simulink model "Stromsensor_three_fase"  (R2020b)
settings: Solver=VariableStepAuto  StartTime=0.0  StopTime=1/60*2  RelTol=1e-3
libraries: fl_lib x27, nesl_utility x9, ee_lib x3
settings Model: Creator=jenel  LastModifiedBy=jenel

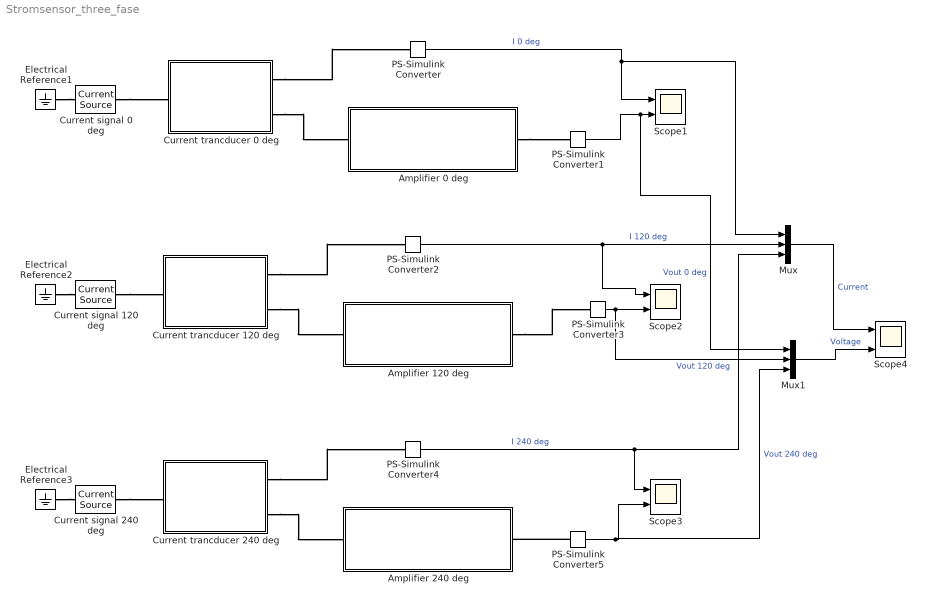
== system Stromsensor_three_fase ==
  Amplifier 0 deg : Subsystem
  Amplifier 120 deg : Subsystem
  Amplifier 240 deg : Subsystem
  Current signal 0 deg : ee_lib/Sources/Current Source  dc_current=0 A  ac_current=200 mA  ac_shift=0 deg  ac_frequency=60 Hz  noise_mode=0  PSD=0 A^2/Hz  repeatability=1  auto_seed=961264961  user_seed=0  sample_time=1e-3 s  i_specify=off  i_priority=None  i=0 A  i_nominal_specify=off  i_nominal_unit=A  i_nominal_value=1  v_specify=off  v_priority=None  v=0 V  v_nominal_specify=off  v_nominal_unit=V  v_nominal_value=1
      settings: SourceProductBaseCode=PS
  Current signal 120 deg : ee_lib/Sources/Current Source  dc_current=0 A  ac_current=200 mA  ac_shift=120 deg  ac_frequency=60 Hz  noise_mode=0  PSD=0 A^2/Hz  repeatability=1  auto_seed=3499211588  user_seed=0  sample_time=1e-3 s  i_specify=off  i_priority=None  i=0 A  i_nominal_specify=off  i_nominal_unit=A  i_nominal_value=1  v_specify=off  v_priority=None  v=0 V  v_nominal_specify=off  v_nominal_unit=V  v_nominal_value=1
      settings: SourceProductBaseCode=PS
  Current signal 240 deg : ee_lib/Sources/Current Source  dc_current=0 A  ac_current=200 mA  ac_shift=240 deg  ac_frequency=60 Hz  noise_mode=0  PSD=0 A^2/Hz  repeatability=1  auto_seed=3890346746  user_seed=0  sample_time=1e-3 s  i_specify=off  i_priority=None  i=0 A  i_nominal_specify=off  i_nominal_unit=A  i_nominal_value=1  v_specify=off  v_priority=None  v=0 V  v_nominal_specify=off  v_nominal_unit=V  v_nominal_value=1
      settings: SourceProductBaseCode=PS
  Current trancducer 0 deg : Subsystem
  Current trancducer 120 deg : Subsystem
  Current trancducer 240 deg : Subsystem
  Electrical Reference1 : fl_lib/Electrical/Electrical Elements/Electrical Reference
  Electrical Reference2 : fl_lib/Electrical/Electrical Elements/Electrical Reference
  Electrical Reference3 : fl_lib/Electrical/Electrical Elements/Electrical Reference
  Mux : Mux  Inputs=3
  Mux1 : Mux  Inputs=3
  PS-Simulink Converter{,1..5} (6 alike) : nesl_utility/PS-Simulink Converter  PhysicalDomain=network_engine_domain  SubClassName=ps_output  LeftPortType=input  RightPortType=output  PseudoPeriodic=off  Frequencies=[]  Unit=inherit  AffineConversion=off
  Scope{1..4} (4 alike) : Scope  NumInputPorts=2
  wires:
  PS-Simulink Converter/1 -> Mux/1, Scope1/1  "I 0 deg"
  PS-Simulink Converter1/1 -> Mux1/1, Scope1/2  "Vout 0 deg"
  PS-Simulink Converter3/1 -> Mux1/2, Scope2/2  "Vout 120 deg"
  PS-Simulink Converter2/1 -> Scope2/1, Mux/2  "I 120 deg"
  PS-Simulink Converter4/1 -> Mux/3, Scope3/1  "I 240 deg"
  PS-Simulink Converter5/1 -> Mux1/3, Scope3/2  "Vout 240 deg"
  Mux/1 -> Scope4/1  "Current"
  Mux1/1 -> Scope4/2  "Voltage"
  connections:
  Current trancducer 0 deg/RConn1 -- PS-Simulink Converter/LConn1
  Electrical Reference1/LConn1 -- Current signal 0 deg/RConn1
  Current signal 0 deg/LConn1 -- Current trancducer 0 deg/LConn1
  Current trancducer 0 deg/RConn2 -- Amplifier 0 deg/LConn1
  Amplifier 0 deg/RConn1 -- PS-Simulink Converter1/LConn1
  Current trancducer 120 deg/RConn2 -- Amplifier 120 deg/LConn1
  Current signal 120 deg/LConn1 -- Current trancducer 120 deg/LConn1
  Amplifier 120 deg/RConn1 -- PS-Simulink Converter3/LConn1
  Electrical Reference2/LConn1 -- Current signal 120 deg/RConn1
  Current trancducer 120 deg/RConn1 -- PS-Simulink Converter2/LConn1
  Current trancducer 240 deg/RConn1 -- PS-Simulink Converter4/LConn1
  Electrical Reference3/LConn1 -- Current signal 240 deg/RConn1
  PS-Simulink Converter5/LConn1 -- Amplifier 240 deg/RConn1
  Current signal 240 deg/LConn1 -- Current trancducer 240 deg/LConn1
  Current trancducer 240 deg/RConn2 -- Amplifier 240 deg/LConn1

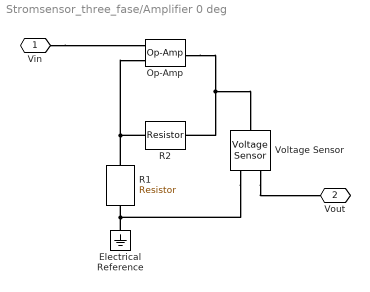
== system Stromsensor_three_fase/Amplifier 0 deg ==
  Electrical Reference : fl_lib/Electrical/Electrical Elements/Electrical Reference
  Op-Amp : fl_lib/Electrical/Electrical Elements/Op-Amp  outI_specify=on  outI_priority=None  outI=0 A  outI_nominal_specify=off  outI_nominal_unit=A  outI_nominal_value=1
  R1 : fl_lib/Electrical/Electrical Elements/Resistor  R=1000 Ohm  i_specify=off  i_priority=None  i=0 A  i_nominal_specify=off  i_nominal_unit=A  i_nominal_value=1  v_specify=off  v_priority=None  v=0 V  v_nominal_specify=off  v_nominal_unit=V  v_nominal_value=1
  R2 : fl_lib/Electrical/Electrical Elements/Resistor  R=666.6667 Ohm  i_specify=off  i_priority=None  i=0 A  i_nominal_specify=off  i_nominal_unit=A  i_nominal_value=1  v_specify=off  v_priority=None  v=0 V  v_nominal_specify=off  v_nominal_unit=V  v_nominal_value=1
  Voltage Sensor : fl_lib/Electrical/Electrical Sensors/Voltage Sensor
  Vin : PMIOPort  Side=Left
  Vout : PMIOPort  Port=2  Side=Right
  connections:
  Op-Amp/RConn1 -- Voltage Sensor/LConn1 -- R2/RConn1
  Vin/RConn1 -- Op-Amp/LConn1
  Electrical Reference/LConn1 -- Voltage Sensor/RConn2 -- R1/RConn1
  R2/LConn1 -- R1/LConn1 -- Op-Amp/LConn2
  Voltage Sensor/RConn1 -- Vout/RConn1

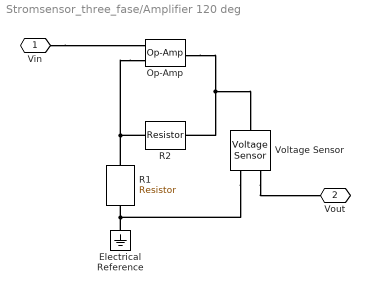
== system Stromsensor_three_fase/Amplifier 120 deg ==
  Electrical Reference : fl_lib/Electrical/Electrical Elements/Electrical Reference
  Op-Amp : fl_lib/Electrical/Electrical Elements/Op-Amp  outI_specify=on  outI_priority=None  outI=0 A  outI_nominal_specify=off  outI_nominal_unit=A  outI_nominal_value=1
  R1 : fl_lib/Electrical/Electrical Elements/Resistor  R=1000 Ohm  i_specify=off  i_priority=None  i=0 A  i_nominal_specify=off  i_nominal_unit=A  i_nominal_value=1  v_specify=off  v_priority=None  v=0 V  v_nominal_specify=off  v_nominal_unit=V  v_nominal_value=1
  R2 : fl_lib/Electrical/Electrical Elements/Resistor  R=666.6667 Ohm  i_specify=off  i_priority=None  i=0 A  i_nominal_specify=off  i_nominal_unit=A  i_nominal_value=1  v_specify=off  v_priority=None  v=0 V  v_nominal_specify=off  v_nominal_unit=V  v_nominal_value=1
  Voltage Sensor : fl_lib/Electrical/Electrical Sensors/Voltage Sensor
  Vin : PMIOPort  Side=Left
  Vout : PMIOPort  Port=2  Side=Right
  connections:
  Voltage Sensor/RConn1 -- Vout/RConn1
  Op-Amp/LConn2 -- R1/LConn1 -- R2/LConn1
  Voltage Sensor/RConn2 -- R1/RConn1 -- Electrical Reference/LConn1
  Vin/RConn1 -- Op-Amp/LConn1
  R2/RConn1 -- Voltage Sensor/LConn1 -- Op-Amp/RConn1

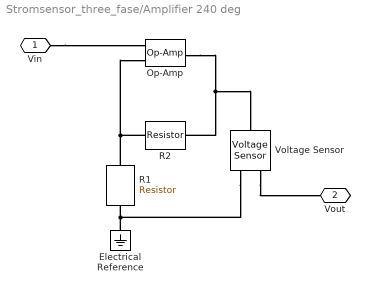
== system Stromsensor_three_fase/Amplifier 240 deg ==
  Electrical Reference : fl_lib/Electrical/Electrical Elements/Electrical Reference
  Op-Amp : fl_lib/Electrical/Electrical Elements/Op-Amp  outI_specify=on  outI_priority=None  outI=0 A  outI_nominal_specify=off  outI_nominal_unit=A  outI_nominal_value=1
  R1 : fl_lib/Electrical/Electrical Elements/Resistor  R=1000 Ohm  i_specify=off  i_priority=None  i=0 A  i_nominal_specify=off  i_nominal_unit=A  i_nominal_value=1  v_specify=off  v_priority=None  v=0 V  v_nominal_specify=off  v_nominal_unit=V  v_nominal_value=1
  R2 : fl_lib/Electrical/Electrical Elements/Resistor  R=666.6667 Ohm  i_specify=off  i_priority=None  i=0 A  i_nominal_specify=off  i_nominal_unit=A  i_nominal_value=1  v_specify=off  v_priority=None  v=0 V  v_nominal_specify=off  v_nominal_unit=V  v_nominal_value=1
  Voltage Sensor : fl_lib/Electrical/Electrical Sensors/Voltage Sensor
  Vin : PMIOPort  Side=Left
  Vout : PMIOPort  Port=2  Side=Right
  connections:
  Op-Amp/RConn1 -- Voltage Sensor/LConn1 -- R2/RConn1
  Vin/RConn1 -- Op-Amp/LConn1
  Electrical Reference/LConn1 -- R1/RConn1 -- Voltage Sensor/RConn2
  R2/LConn1 -- R1/LConn1 -- Op-Amp/LConn2
  Voltage Sensor/RConn1 -- Vout/RConn1

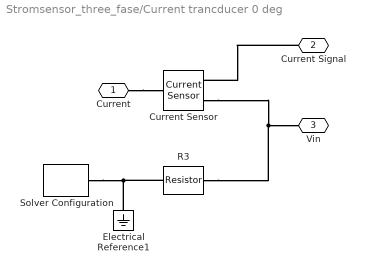
== system Stromsensor_three_fase/Current trancducer 0 deg ==
  Current Sensor : fl_lib/Electrical/Electrical Sensors/Current Sensor
  Electrical Reference1 : fl_lib/Electrical/Electrical Elements/Electrical Reference
  R3 : fl_lib/Electrical/Electrical Elements/Resistor  R=30 Ohm  i_specify=off  i_priority=None  i=0 A  i_nominal_specify=off  i_nominal_unit=A  i_nominal_value=1  v_specify=off  v_priority=None  v=0 V  v_nominal_specify=off  v_nominal_unit=V  v_nominal_value=1
  Solver Configuration : nesl_utility/Solver Configuration  PhysicalDomain=network_engine_domain  SubClassName=solver  LeftPortType=input  RightPortType=generic  Tones=[]  Harmonics=[]  SimulateNoise=off  Profile=off  UseLocalSampling=off  EnableSwitchedLinearOptims=on  FrequencyDomain=off  UseCCode=off  RelTol=0.001  AbsTol=1e-06  MinStep=1e-09  ToWorkspace=off  RevertToSquareIcSolve=off  NumHomotopyIterations=100  PhasorMode=off  PhasorModeNumHarmonics=1  DoDC=off  ResidualTolerance=1e-09  UseLocalSolver=off  LocalSolverChoice=NE_BACKWARD_EULER_ADVANCER  LocalSolverSampleTime=0.001  DoFixedCost=off  MaxNonlinIter=3  MaxModeIter=2  ComputeImpulses=off  ImpulseIterations=2  LinearAlgebra=auto  EquationFormulation=NE_TIME_EF  DelaysMemoryBudget=1024  AutomaticFiltering=on  FilteringTimeConstant=0.001  PartitionStorageMethod=AS_NEEDED  PartitionMemoryBudget=1024  PartitionMethod=ROBUST
  Current : PMIOPort  Side=Left
  Current Signal : PMIOPort  Port=2  Side=Right
  Vin : PMIOPort  Port=3  Side=Right
  connections:
  Current/RConn1 -- Current Sensor/LConn1
  Current Signal/RConn1 -- Current Sensor/RConn1
  Current Sensor/RConn2 -- Vin/RConn1 -- R3/LConn1
  Electrical Reference1/LConn1 -- Solver Configuration/RConn1 -- R3/RConn1

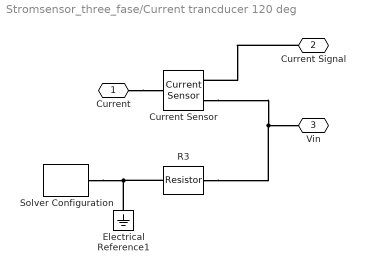
== system Stromsensor_three_fase/Current trancducer 120 deg ==
  Current Sensor : fl_lib/Electrical/Electrical Sensors/Current Sensor
  Electrical Reference1 : fl_lib/Electrical/Electrical Elements/Electrical Reference
  R3 : fl_lib/Electrical/Electrical Elements/Resistor  R=30 Ohm  i_specify=off  i_priority=None  i=0 A  i_nominal_specify=off  i_nominal_unit=A  i_nominal_value=1  v_specify=off  v_priority=None  v=0 V  v_nominal_specify=off  v_nominal_unit=V  v_nominal_value=1
  Solver Configuration : nesl_utility/Solver Configuration  PhysicalDomain=network_engine_domain  SubClassName=solver  LeftPortType=input  RightPortType=generic  Tones=[]  Harmonics=[]  SimulateNoise=off  Profile=off  UseLocalSampling=off  EnableSwitchedLinearOptims=on  FrequencyDomain=off  UseCCode=off  RelTol=0.001  AbsTol=1e-06  MinStep=1e-09  ToWorkspace=off  RevertToSquareIcSolve=off  NumHomotopyIterations=100  PhasorMode=off  PhasorModeNumHarmonics=1  DoDC=off  ResidualTolerance=1e-09  UseLocalSolver=off  LocalSolverChoice=NE_BACKWARD_EULER_ADVANCER  LocalSolverSampleTime=0.001  DoFixedCost=off  MaxNonlinIter=3  MaxModeIter=2  ComputeImpulses=off  ImpulseIterations=2  LinearAlgebra=auto  EquationFormulation=NE_TIME_EF  DelaysMemoryBudget=1024  AutomaticFiltering=on  FilteringTimeConstant=0.001  PartitionStorageMethod=AS_NEEDED  PartitionMemoryBudget=1024  PartitionMethod=ROBUST
  Current : PMIOPort  Side=Left
  Current Signal : PMIOPort  Port=2  Side=Right
  Vin : PMIOPort  Port=3  Side=Right
  connections:
  R3/RConn1 -- Solver Configuration/RConn1 -- Electrical Reference1/LConn1
  R3/LConn1 -- Vin/RConn1 -- Current Sensor/RConn2
  Current Signal/RConn1 -- Current Sensor/RConn1
  Current/RConn1 -- Current Sensor/LConn1

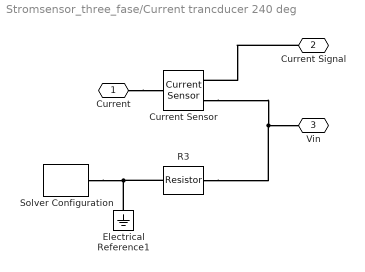
== system Stromsensor_three_fase/Current trancducer 240 deg ==
  Current Sensor : fl_lib/Electrical/Electrical Sensors/Current Sensor
  Electrical Reference1 : fl_lib/Electrical/Electrical Elements/Electrical Reference
  R3 : fl_lib/Electrical/Electrical Elements/Resistor  R=30 Ohm  i_specify=off  i_priority=None  i=0 A  i_nominal_specify=off  i_nominal_unit=A  i_nominal_value=1  v_specify=off  v_priority=None  v=0 V  v_nominal_specify=off  v_nominal_unit=V  v_nominal_value=1
  Solver Configuration : nesl_utility/Solver Configuration  PhysicalDomain=network_engine_domain  SubClassName=solver  LeftPortType=input  RightPortType=generic  Tones=[]  Harmonics=[]  SimulateNoise=off  Profile=off  UseLocalSampling=off  EnableSwitchedLinearOptims=on  FrequencyDomain=off  UseCCode=off  RelTol=0.001  AbsTol=1e-06  MinStep=1e-09  ToWorkspace=off  RevertToSquareIcSolve=off  NumHomotopyIterations=100  PhasorMode=off  PhasorModeNumHarmonics=1  DoDC=off  ResidualTolerance=1e-09  UseLocalSolver=off  LocalSolverChoice=NE_BACKWARD_EULER_ADVANCER  LocalSolverSampleTime=0.001  DoFixedCost=off  MaxNonlinIter=3  MaxModeIter=2  ComputeImpulses=off  ImpulseIterations=2  LinearAlgebra=auto  EquationFormulation=NE_TIME_EF  DelaysMemoryBudget=1024  AutomaticFiltering=on  FilteringTimeConstant=0.001  PartitionStorageMethod=AS_NEEDED  PartitionMemoryBudget=1024  PartitionMethod=ROBUST
  Current : PMIOPort  Side=Left
  Current Signal : PMIOPort  Port=2  Side=Right
  Vin : PMIOPort  Port=3  Side=Right
  connections:
  Current/RConn1 -- Current Sensor/LConn1
  Current Signal/RConn1 -- Current Sensor/RConn1
  Current Sensor/RConn2 -- Vin/RConn1 -- R3/LConn1
  Electrical Reference1/LConn1 -- Solver Configuration/RConn1 -- R3/RConn1
